simulink model "MechanicalMassSpringContinousTime"  (R2021b)
settings: Solver=ode45  StartTime=0.0  StopTime=200  RelTol=1e-3  EnableMultiTasking=on
values from neighbouring files (symbols this model uses):
  Continuous_Plant_Model = ss(A, B, C, D)    [MpcDesignExe1.m]
settings Model: Creator=hg212  LastModifiedBy=wsmur
settings SolverCC: AlgebraicLoopSolver=TrustRegion
settings DataIOCC: LimitDataPoints=on  SaveFormat=Array  ReturnWorkspaceOutputs=off
settings OptimizationCC: LifeSpan=inf
settings DebuggingCC: InheritedTsInSrcMsg=none  SFUnexpectedBacktrackingDiag=warning  SFNoUnconditionalDefaultTransitionDiag=warning  SFExecutionAtInitializationDiag=none  SFMachineParentedDataDiag=warning  ArithmeticOperatorsInVariantConditions=warning
settings HardwareCC: ProdBitPerPointer=32  ProdBitPerSizeT=32  ProdBitPerPtrDiffT=32  ProdLargestAtomicFloat=None  ProdIntDivRoundTo=Undefined  ProdEndianess=Unspecified  ProdWordSize=32  ProdHWDeviceType=32-bit Generic
settings ModelReferenceCC: PropagateSignalLabelsOutOfModel=off
settings SFSimCC: SimUseLocalCustomCode=off  CustomCodeUndefinedFunction=UseInterfaceOnly
settings RTWCC: RTWUseLocalCustomCode=off
settings CodeAppCC: StateflowObjectComments=on
settings GRTTargetCC: TargetLangStandard=C89/C90 (ANSI)
settings ConfigComp: CovMetricSettings=dw  CovSaveCumulativeToWorkspaceVar=on  CovSaveSingleToWorkspaceVar=on  CovExternalEMLEnable=off

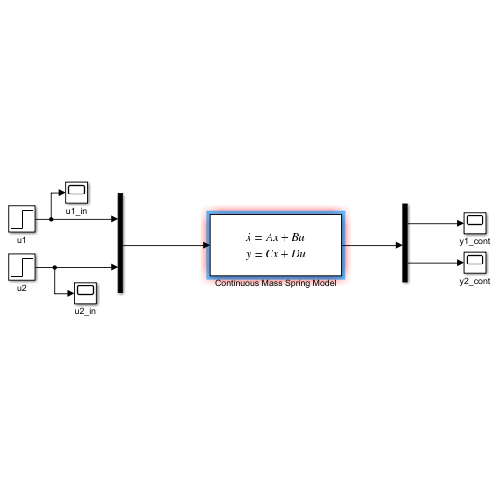
[thumbnail: Simulink's stored preview of the top-level diagram]
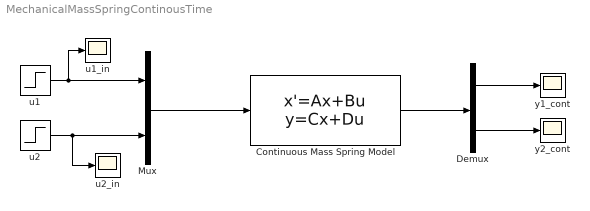
== system MechanicalMassSpringContinousTime ==
  Continuous Mass Spring Model : StateSpace  A=Continuous_Plant_Model.A  B=Continuous_Plant_Model.B  C=Continuous_Plant_Model.C  D=Continuous_Plant_Model.D  InitialCondition=0
  Demux : Demux  Outputs=2
  Mux : Mux  Inputs=2
  u1 : Step  Time=50
  u1_in : Scope
  u2 : Step  Time=150
  u2_in : Scope
  y1_cont : Scope
  y2_cont : Scope
  wires:
  Mux/1 -> Continuous Mass Spring Model/1
  u1/1 -> u1_in/1, Mux/1
  u2/1 -> u2_in/1, Mux/2
  Demux/1 -> y1_cont/1
  Demux/2 -> y2_cont/1
  Continuous Mass Spring Model/1 -> Demux/1
